simulink model "statechart2_2"  (R2016b)
settings: Solver=VariableStepAuto  StartTime=0.0  StopTime=25  MaxStep=0.05  RelTol=1e-3
libraries: dspindex x3
settings Model: Creator=larry  LastModifiedBy=larry

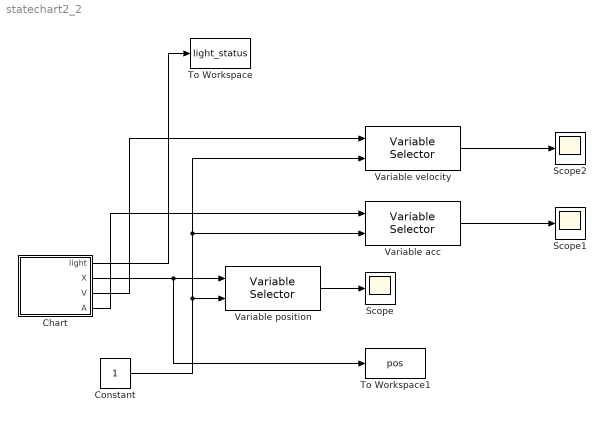
== system statechart2_2 ==
  Chart : Stateflow chart  TreatAsAtomicUnit=on
  Constant : Constant
  Scope : Scope
  Scope1 : Scope
  Scope2 : Scope
  To Workspace : ToWorkspace  VariableName=light_status  SampleTime=-1
  To Workspace1 : ToWorkspace  VariableName=pos  SampleTime=-1
  Variable acc : dspindex/Variable Selector  NumInputs=1  rowsOrCols=Columns  IdxMode=Variable  Elements=[1 3]  ZerOneIdxMode=One-based  errmode=Clip Index  FillMode=on  FillValues=0
  Variable position : dspindex/Variable Selector  NumInputs=1  rowsOrCols=Columns  IdxMode=Variable  Elements=[1 3]  ZerOneIdxMode=One-based  errmode=Clip Index  FillMode=on  FillValues=0
  Variable velocity : dspindex/Variable Selector  NumInputs=1  rowsOrCols=Columns  IdxMode=Variable  Elements=[1 3]  ZerOneIdxMode=One-based  errmode=Clip Index  FillMode=on  FillValues=0
  wires:
  Chart/1(light) -> To Workspace/1
  Chart/2(X) -> To Workspace1/1, Variable position/1
  Constant/1 -> Variable acc/2, Variable velocity/2, Variable position/2
  Variable position/1 -> Scope/1
  Variable acc/1 -> Scope1/1
  Variable velocity/1 -> Scope2/1
  Chart/3(V) -> Variable velocity/1
  Chart/4(A) -> Variable acc/1

== stateflow chart statechart2_2/Chart ==
  state Light [parallel]
    settings: executionOrder=1
    state Y_R
      en:
      light = 4;
    state R_G
      en:
      light = 1;
    state G_R
      en:
      light = 3;
    state R_Y
      en:
      light = 2;
    G_R -> Y_R : after(2.5, sec)
    Y_R -> R_G : after(0.5, sec)
    (default) -> R_G
    R_Y -> G_R : after(0.5, sec)
    R_G -> R_Y : after(2.5, sec)
  state agent0 [parallel]
    settings: executionOrder=2
    state Straight
      state FreeDriving
        state AccFromStop
          en:
          A(this,:) = [A_MAX, 0];
          du:
          accDrive(this);
        state Acc
          en:
          A(this,:) = [0.5*A_MAX, 0];
          du:
          accDrive(this);
        state FixRate
          en:
          A(this,:) = [0, 0];
          fixRate(this, V_MAX);
          du:
          fixRateDrive(this);
        (default) -> (junction 71)
        (junction 71) -> agent0.Straight.FreeDriving.AccFromStop [order 2]
        (junction 71) -> (junction 299) [order 1] : [~isStopped(this)]
        agent0.Straight.FreeDriving.AccFromStop -> agent0.Straight.FreeDriving.Acc : [reachRate(this, 3.0/5*V_MAX)]
        (junction 299) -> agent0.Straight.FreeDriving.Acc [order 2]
        (junction 299) -> agent0.Straight.FreeDriving.FixRate [order 1] : [reachRate(this, V_MAX)]
        agent0.Straight.FreeDriving.Acc -> agent0.Straight.FreeDriving.FixRate : [reachRate(this, V_MAX)]
      state Follow
        du:
        followFrontCar(this, A_MAX);
      (default) -> agent0.Straight.FreeDriving
      agent0.Straight.FreeDriving -> agent0.Straight.Follow : [hasFrontCar(this)]
      agent0.Straight.Follow -> agent0.Straight.FreeDriving : [~hasFrontCar(this)]
    state IDLE
    state SlowToStop
      state SlowDown
        en:
        updateBrakeAcc(this, A_MAX, stop);
        du:
        accDrive(this);
      state Stopped
        en:
        A(this,:) = [0, 0];
        V(this,:) = [0, 0];
      (default) -> agent0.SlowToStop.SlowDown
      agent0.SlowToStop.SlowDown -> Stopped : [isStopped(this)]
    (default) -> agent0.Straight [order 1] : [enabled]
    (default) -> agent0.IDLE [order 2]
    agent0.SlowToStop -> agent0.Straight : [in(Light.G_R)]
    (junction 1589) -> agent0.SlowToStop
    (junction 1588) -> (junction 1589) [order 1] : [hasFrontCar(this)]...
        | {stop = getStopPos(this, INTER)}
    agent0.Straight -> (junction 1588) : [in(Light.R_G) &&...
        | closeTo(this,INTER)]
    (junction 1590) -> (junction 1589) [order 1] : [isStoppable(this,A_MAX,INTER)]...
        | {stop = INTER}
    (junction 1588) -> (junction 1590) [order 2]
    (junction 1590) -> agent0.Straight [order 2]
  state Vehicle2 [parallel]
    settings: executionOrder=4
    state Straight
      state FreeDriving
        state AccFromStop
          en:
          A(this,:) = [A_MAX, 0];
          du:
          accDrive(this);
        state Acc
          en:
          A(this,:) = [0.5*A_MAX, 0];
          du:
          accDrive(this);
        state FixRate
          en:
          A(this,:) = [0, 0];
          fixRate(this, V_MAX);
          du:
          fixRateDrive(this);
        (default) -> (junction 2261)
        (junction 2261) -> Vehicle2.Straight.FreeDriving.AccFromStop [order 2]
        (junction 2261) -> (junction 2262) [order 1] : [~isStopped(this)]
        Vehicle2.Straight.FreeDriving.AccFromStop -> Vehicle2.Straight.FreeDriving.Acc : [reachRate(this, 3.0/5*V_MAX)]
        (junction 2262) -> Vehicle2.Straight.FreeDriving.Acc [order 2]
        (junction 2262) -> Vehicle2.Straight.FreeDriving.FixRate [order 1] : [reachRate(this, V_MAX)]
        Vehicle2.Straight.FreeDriving.Acc -> Vehicle2.Straight.FreeDriving.FixRate : [reachRate(this, V_MAX)]
      state Follow
        du:
        followFrontCar(this, A_MAX);
      (default) -> Vehicle2.Straight.FreeDriving
      Vehicle2.Straight.FreeDriving -> Vehicle2.Straight.Follow : [hasFrontCar(this)]
      Vehicle2.Straight.Follow -> Vehicle2.Straight.FreeDriving : [~hasFrontCar(this)]
    state RoadIntersection
      state Follow
        state Adjust
          du:
          adjustBehind(this, X(front,:), 0.5*SAFE_DIST);
        state FollowFront
          du:
          followFrontCar(this, A_MAX);
        state SlowDown
          en:
          updateBrakeAcc(this,A_MAX, ...
          getStopPos(this,INTER));
          du:
          accDrive(this);
        (default) -> Vehicle2.RoadIntersection.Follow.FollowFront [order 1] : [in(Light.G_R)]
        Vehicle2.RoadIntersection.Follow.SlowDown -> Vehicle2.RoadIntersection.Follow.Adjust : [isStopped(this)]
        Vehicle2.RoadIntersection.Follow.FollowFront -> Vehicle2.RoadIntersection.Follow.SlowDown : [in(Light.Y_R)]
        (default) -> Vehicle2.RoadIntersection.Follow.SlowDown [order 2]
      state FreeDriving
        state SlowToStop
          state SlowDown
            en:
            updateBrakeAcc(this,A_MAX, INTER);
            du:
            accDrive(this);
          state Stop
            en:
            A(this,:) = [0, 0];
            V(this,:) = [0, 0];
          state Adjust
            en:
            fixRate(this,V_MIN);
            du:
            adjustBehind(this,INTER,...
            0.5*SAFE_DIST);
          (default) -> Vehicle2.RoadIntersection.FreeDriving.SlowToStop.SlowDown
          Vehicle2.RoadIntersection.FreeDriving.SlowToStop.SlowDown -> Vehicle2.RoadIntersection.FreeDriving.SlowToStop.Stop : [isStopped(this)]
          Vehicle2.RoadIntersection.FreeDriving.SlowToStop.Adjust -> Vehicle2.RoadIntersection.FreeDriving.SlowToStop.Stop : [isStopped(this)]
          Vehicle2.RoadIntersection.FreeDriving.SlowToStop.Stop -> Vehicle2.RoadIntersection.FreeDriving.SlowToStop.Adjust : [closeBehind(this,INTER,...
              | 0.5*SAFE_DIST)]
        state FixRate
          en:
          A(this,:) = [0, 0];
          du:
          fixRateDrive(this);
        state AccFromStop
          en:
          A(this,:) = [A_MAX, 0];
          du:
          accDrive(this);
        (default) -> Vehicle2.RoadIntersection.FreeDriving.SlowToStop [order 2]
        (default) -> Vehicle2.RoadIntersection.FreeDriving.FixRate [order 1] : [in(Light.G_R)]
        Vehicle2.RoadIntersection.FreeDriving.FixRate -> (junction 2288) : [in(Light.Y_R)]
        (junction 2288) -> Vehicle2.RoadIntersection.FreeDriving.SlowToStop [order 1] : [isStoppable(this,A_MAX,INTER)]
        (junction 2288) -> Vehicle2.RoadIntersection.FreeDriving.AccFromStop [order 2]
        Vehicle2.RoadIntersection.FreeDriving.SlowToStop -> Vehicle2.RoadIntersection.FreeDriving.AccFromStop : [in(Light.G_R)]
      (default) -> Vehicle2.RoadIntersection.Follow [order 1] : [hasFrontCar(this)]
      Vehicle2.RoadIntersection.FreeDriving -> Vehicle2.RoadIntersection.Follow : [hasFrontCar(this)]
      Vehicle2.RoadIntersection.Follow -> Vehicle2.RoadIntersection.FreeDriving : [~hasFrontCar(this)]
      (default) -> Vehicle2.RoadIntersection.FreeDriving [order 2]
    state IDLE
    (default) -> Vehicle2.Straight [order 1] : [enabled]
    Vehicle2.RoadIntersection -> Vehicle2.Straight : [~closeTo(this,INTER)]
    Vehicle2.Straight -> Vehicle2.RoadIntersection : [closeTo(this,INTER)]
    (default) -> Vehicle2.IDLE [order 2]
  state Vehicle1 [parallel]
    settings: executionOrder=3
    state Straight
      state FreeDriving
        state AccFromStop
          en:
          A(this,:) = [A_MAX, 0];
          du:
          accDrive(this);
        state Acc
          en:
          A(this,:) = [0.5*A_MAX, 0];
          du:
          accDrive(this);
        state FixRate
          en:
          A(this,:) = [0, 0];
          fixRate(this, V_MAX);
          du:
          fixRateDrive(this);
        (default) -> (junction 1992)
        (junction 1992) -> Vehicle1.Straight.FreeDriving.AccFromStop [order 2]
        (junction 1992) -> (junction 1993) [order 1] : [~isStopped(this)]
        Vehicle1.Straight.FreeDriving.AccFromStop -> Vehicle1.Straight.FreeDriving.Acc : [reachRate(this, 3.0/5*V_MAX)]
        (junction 1993) -> Vehicle1.Straight.FreeDriving.Acc [order 2]
        (junction 1993) -> Vehicle1.Straight.FreeDriving.FixRate [order 1] : [reachRate(this, V_MAX)]
        Vehicle1.Straight.FreeDriving.Acc -> Vehicle1.Straight.FreeDriving.FixRate : [reachRate(this, V_MAX)]
      state Follow
        en:
        front = getFrontCarIdx(this);
        du:
        followFrontCar(this, A_MAX);
      (default) -> Vehicle1.Straight.FreeDriving
      Vehicle1.Straight.FreeDriving -> Vehicle1.Straight.Follow : [hasFrontCar(this)]
      Vehicle1.Straight.Follow -> Vehicle1.Straight.FreeDriving : [~hasFrontCar(this)]
    state RoadIntersection
      state Follow
        en:
        front = getFrontCarIdx(this);
        state FollowFront
          du:
          followFrontCar(this, A_MAX);
        state SlowToStop
          state SlowDown
            en:
            updateBrakeAcc(this,A_MAX, ...
            closestObj(this,INTER,X(front,:)));
            du:
            accDrive(this);
          state Adjust
            du:
            adjustBehind(this, X(front,:), ...
            SAFE_DIST);
          (default) -> Vehicle1.RoadIntersection.Follow.SlowToStop.SlowDown
          Vehicle1.RoadIntersection.Follow.SlowToStop.SlowDown -> Vehicle1.RoadIntersection.Follow.SlowToStop.Adjust : [isStopped(this)]
        (default) -> Vehicle1.RoadIntersection.Follow.FollowFront [order 1] : [in(Light.G_R)]
        (junction 2312) -> Vehicle1.RoadIntersection.Follow.FollowFront [order 2]
        (default) -> (junction 2312) [order 2]
        Vehicle1.RoadIntersection.Follow.FollowFront -> (junction 2312) : [in(Light.Y_R)]
        (junction 2312) -> Vehicle1.RoadIntersection.Follow.SlowToStop [order 1] : [isStoppable(this, A_MAX,...
            | closestObj(this, INTER,X(front,:)))]
        Vehicle1.RoadIntersection.Follow.SlowToStop -> Vehicle1.RoadIntersection.Follow.FollowFront : [in(Light.G_R)]
      state FreeDriving
        state FixRate
          en:
          A(this,:) = [0, 0];
          du:
          fixRateDrive(this);
        state SlowToStop
          state SlowDown
            en:
            updateBrakeAcc(this,A_MAX, INTER);
            du:
            accDrive(this);
          state Stop
            en:
            A(this,:) = [0, 0];
            V(this,:) = [0, 0];
          state Adjust
            en:
            fixRate(this,V_MIN);
            du:
            adjustBehind(this,INTER,...
            SAFE_DIST);
          (default) -> Vehicle1.RoadIntersection.FreeDriving.SlowToStop.SlowDown
          Vehicle1.RoadIntersection.FreeDriving.SlowToStop.SlowDown -> Vehicle1.RoadIntersection.FreeDriving.SlowToStop.Stop : [isStopped(this)]
          Vehicle1.RoadIntersection.FreeDriving.SlowToStop.Adjust -> Vehicle1.RoadIntersection.FreeDriving.SlowToStop.Stop : [isStopped(this)]
          Vehicle1.RoadIntersection.FreeDriving.SlowToStop.Stop -> Vehicle1.RoadIntersection.FreeDriving.SlowToStop.Adjust : [closeBehind(this,INTER,...
              | SAFE_DIST)]
        state AccFromStop
          en:
          A(this,:) = [A_MAX, 0];
          du:
          accDrive(this);
        (default) -> Vehicle1.RoadIntersection.FreeDriving.FixRate [order 1] : [in(Light.G_R)]
        Vehicle1.RoadIntersection.FreeDriving.FixRate -> (junction 2062) : [in(Light.Y_R)]
        (default) -> (junction 2062) [order 2]
        (junction 2062) -> Vehicle1.RoadIntersection.FreeDriving.SlowToStop [order 1] : [isStoppable(this,A_MAX,INTER)]
        (junction 2062) -> Vehicle1.RoadIntersection.FreeDriving.AccFromStop [order 2]
        Vehicle1.RoadIntersection.FreeDriving.SlowToStop -> Vehicle1.RoadIntersection.FreeDriving.AccFromStop : [in(Light.G_R)]
      (default) -> Vehicle1.RoadIntersection.Follow [order 1] : [hasFrontCar(this)]
      Vehicle1.RoadIntersection.FreeDriving -> Vehicle1.RoadIntersection.Follow : [hasFrontCar(this)]
      Vehicle1.RoadIntersection.Follow -> Vehicle1.RoadIntersection.FreeDriving : [~hasFrontCar(this)]
      (default) -> Vehicle1.RoadIntersection.FreeDriving [order 2]
    state IDLE
    (default) -> Vehicle1.Straight [order 1] : [enabled]
    Vehicle1.RoadIntersection -> Vehicle1.Straight : [~closeTo(this,INTER)]
    Vehicle1.Straight -> Vehicle1.RoadIntersection : [closeTo(this,INTER)]
    (default) -> Vehicle1.IDLE [order 2]
  data: self function_input; obj1 function_input; pos function_output; obj2 function_input; self function_input; obj function_input; pos function_output; self function_input; amax function_input; obj function_input; self function_input; res function_output; self function_input; amax function_input; obj function_input; res function_output; self function_input; amax function_input; self function_input; res function_output; self function_input; idx function_output; self function_input; res function_output; obj function_input; this constant uint8 size=1 =1; V_MAX constant double size=1 =2.5; A_MAX constant double size=1 =2.5; stop local double size=[1, 2] =[0, 0]; INTER local double size=[1, 2] =[-1, -0.5]; enabled local boolean size=1 =false; self function_input; rate function_input; res function_output; this constant uint8 size=1 =2; V_MAX constant double size=1 =2.5; A_MAX constant double size=1 =2.5; INTER local double size=[1, 2] =[-1, -0.5]; enabled local boolean size=1 =true; front local uint8 size=1 =uint8(0); self function_input; rate function_input; self function_input; this constant uint8 size=1 =1; V_MAX constant double size=1 =2.5; A_MAX constant double size=1 =2.5; INTER local double size=[1, 2] =[-1, -0.5]; enabled local boolean size=1 =true; front local uint8 size=1 =uint8(0); self function_input; self function_input; obj function_input; dist function_input; res function_output; self function_input; pos function_input; dist function_input; dt constant double size=1 =0.05; light output size=1; WORLD_SIZE constant double size=1 =8; X output size=[2,2] =[-7 -0.5;-6 -0.5]; D local size=[2,2] =[1 0;1 0]; SAFE_DIST constant double size=1 =1; V output size=[2,2] =[0 0;0 0]; A output size=[2,2] =[0 0;0 0]; V_MIN constant double size=1 =0.25
  function pos = closestObj(self, obj1, obj2):
    | function pos = closestObj(self, obj1, obj2)
    | 
    | x = X(self, :);
    | d = D(self, :);
    | 
    | offset = 2*WORLD_SIZE;
    | dX = zeros(2, 1);
    | dX(1) = mod(dot(obj1 - x, d) + offset, offset);
    | dX(2) = mod(dot(obj2 - x, d) + offset, offset);
    | 
    | [~, index] = min(dX);
    | if index == 1
    |     pos = obj1;
    | else
    |     pos = obj2;
    | end
  function pos = getStopPos(self, obj):
    | function pos = getStopPos(self, obj)
    | 
    | dX = zeros(size(X, 1), 1);
    | x = X(self,:);
    | d = D(self,:);
    | 
    | for k=1:length(dX)
    |     dX(k) = dot(X(k,:) - x, d);
    |     if dX(k) < 0
    |         dX(k) = dX(k) + 2*WORLD_SIZE;
    |     end
    | end
    | 
    | % set zero dX to a large enough value
    | dX(dX == 0) = 100;
    | [frontDist, index] = min(dX);
    | interDist = dot(obj - x, d);
    | 
    | if frontDist < interDist
    |     pos = X(index, :);
    | else
    |     pos = obj;
    | end
  function updateBrakeAcc(self, amax, obj):
    | function updateBrakeAcc(self, amax, obj)
    | 
    | x = X(self, :);
    | v = V(self, :);
    | 
    | % add safe distance
    | dist = norm(obj - x) - SAFE_DIST;
    | 
    | assert(dist >= 0);
    | 
    | vnorm = norm(v);
    | reverse = v/vnorm*(-1);
    | a = reverse*vnorm*vnorm/2/dist;
    | anorm = norm(a);
    | 
    | if(anorm >= amax)
    |     a = a/anorm*amax;
    | end
    | 
    | A(self, :) = a;
  function res = hasFrontCar(self):
    | function res = hasFrontCar(self)
    | 
    | 
    | res = false;
    | num = size(X, 1);
    | if num == 1
    |     return;
    | end
    | 
    | dX = zeros(num, 1);
    | x = X(self,:);
    | d = D(self,:);
    | for k=1:length(dX)
    |     dX(k) = dot(X(k,:) - x, d);
    |     if dX(k) < 0
    |         dX(k) = dX(k) + 2*WORLD_SIZE;
    |     end
    | end
    | 
    | % set zero dX to a large enough value
    | dX(dX == 0) = 100;
    | close = min(dX);
    | 
    | if close <= 2*SAFE_DIST
    |     res = true;
    | end
  function res = isStoppable(self, amax, obj):
    | function res = isStoppable(self, amax, obj)
    | 
    | x = X(self, :);
    | v = V(self, :);
    | dist = norm(obj - x) - SAFE_DIST;
    | 
    | vnorm = norm(v);
    | brake_dist = vnorm*vnorm/2.0/amax;
    | res = (brake_dist <= dist);
  function followFrontCar(self, amax):
    | function followFrontCar(self, amax)
    | 
    | dX = zeros(size(X, 1), 1);
    | x = X(self,:);
    | v = V(self,:);
    | d = D(self,:);
    | a = [0, 0];
    | 
    | for k=1:length(dX)
    |     dX(k) = dot(X(k,:) - x, d);
    |     if dX(k) < 0
    |         dX(k) = dX(k) + 2*WORLD_SIZE;
    |     end
    | end
    | 
    | % set zero dX to a large enough value
    | dX(dX == 0) = 100;
    | [dist, idx] = min(dX);
    | 
    | % there must be only one vehicle in front of target agent
    | assert(length(idx) == 1);
    | vo = V(idx(1), :);
    | 
    | if dist <= 2*SAFE_DIST
    |     
    |     if dist <= 1.5*SAFE_DIST
    |         vo = 0.75*vo;
    |     elseif dist <= SAFE_DIST
    |         vo = 0.5*vo;
    |     end
    |     
    |     ar = (vo - v) / dt;
    |     arnorm = norm(ar);
    |     if arnorm > amax
    |         ar = ar/arnorm * amax;
    |         x = x + v * dt + 0.5 * ar * dt * dt;
    |         v = v + ar * dt;
    |     else
    |         x = x + (v + vo) * dt / 2;
    |         v = vo;
    |     end
    |     a = ar;
    |     
    |     % a rounded world
    |     if x(1) > WORLD_SIZE
    |         x(1) = -WORLD_SIZE;
    |     elseif x(1) < -WORLD_SIZE
    |         x(1) = WORLD_SIZE;
    |     end
    | else
    |     assert(false);
    | end
    | 
    | 
    | X(self,:) = x;
    | V(self,:) = v;
    | A(self,:) = a;
  function res = isStopped(self):
    | function res = isStopped(self)
    | 
    | v = V(self,:);
    | d = D(self,:);
    | 
    | res = false;
    | if(dot(v, d) <= 0)
    |     res = true;
    | end
    | if norm(v) < V_MIN
    |     res = true;
    | end
  function idx = getFrontCarIdx(self):
    | function idx = getFrontCarIdx(self)
    | 
    | dX = zeros(size(X, 1), 1);
    | x = X(self,:);
    | v = V(self,:);
    | d = D(self,:);
    | 
    | for k=1:length(dX)
    |     dX(k) = dot(X(k,:) - x, d);
    |     if dX(k) < 0
    |         dX(k) = dX(k) + 2*WORLD_SIZE;
    |     end
    | end
    | 
    | % set zero dX to a large enough value
    | dX(dX == 0) = 100;
    | [~, idx] = min(dX);
    | idx = uint8(idx);
  function res = closeTo(self, obj):
    | function res = closeTo(self, obj)
    | 
    | x = X(self, :);
    | d = D(self, :);
    | 
    | res = false;
    | dist = dot(obj - x, d);
    | if dist > 0 && dist <= 2.5*SAFE_DIST
    |     res = true;
    | end
  function res = reachRate(self, rate):
    | function res = reachRate(self, rate)
    | 
    | res = false;
    | if norm(V(self, :)) >= rate
    |     res = true;
    | end
  function fixRate(self, rate):
    | function fixRate(self, rate)
    |  
    | v = V(self, :);
    | d = D(self, :);
    | if norm(v) < V_MIN
    |     v = d * V_MIN;
    | else
    |     v = v/norm(v)*rate;
    | end
    | 
    | V(self, :) = v;
  function fixRateDrive(self):
    | function fixRateDrive(self)
    |  
    | x = X(self, :);
    | v = V(self, :);
    | 
    | x = x + v * dt;
    | 
    | % a rounded world
    | if x(1) > WORLD_SIZE
    |     x(1) = -WORLD_SIZE;
    | elseif x(1) < -WORLD_SIZE
    |     x(1) = WORLD_SIZE;
    | end
    | 
    | X(self, :) = x;
  function accDrive(self):
    | function accDrive(self)
    | 
    | x = X(self, :);
    | v = V(self, :);
    | a = A(self, :);
    | 
    | x = x + v * dt + 0.5 * a * dt * dt;
    | v = v + a * dt;
    | 
    | if x(1) > WORLD_SIZE
    |     x(1) = -WORLD_SIZE;
    | elseif x(1) < -WORLD_SIZE
    |     x(1) = WORLD_SIZE;
    | end
    | 
    | X(self, :) = x;
    | V(self, :) = v;
  function res = closeBehind(self, obj, dist):
    | function res = closeBehind(self, obj, dist)
    | 
    | x = X(self, :);
    | d = D(self, :);
    | 
    | res = false;
    | diff = dot(obj - x, d);
    | if diff > dist && diff - dist <= 1.5*SAFE_DIST
    |     res = true;
    | end
  function adjustBehind(self, pos, dist):
    | function adjustBehind(self, pos, dist)
    | 
    | x = X(self,:);
    | v = V(self,:);
    | d = D(self,:);
    | 
    | assert(norm(v) <= 1);
    | 
    | diff = dot(pos - x, d);
    | if diff > dist
    |     v = v/norm(v)*V_MIN;
    |     dxnorm = V_MIN * dt;
    |     if (diff - dxnorm) >= dist
    |         x = x + dxnorm * d;
    |     else
    |         x = pos - dist * d;
    |     end
    | else
    |     v = [0, 0];
    | end
    | 
    | X(self, :) = x;
    | V(self, :) = v;
